simulink model "dynamicInversionControl"  (R2025a)
settings: Solver=FixedStepAuto  StartTime=0.0  StopTime=100  FixedStep=0.01  MaxStep=0.2  RelTol=1e-3
PreLoadFcn:
  | addpath('utils','userDefined');
InitFcn:
  | initialParameters;
values from neighbouring files (symbols this model uses):
  ics = JsonLoad('initialConditions.json')    [initialParameters.m]
  params = JsonLoad('params.json')    [initialParameters.m]
undefined symbols (not defined in the file or in its folder): sim_
libraries: sharedutil x2, aerolibutil x1, dspinverses x1
CloseFcn:
  | rmpath('utils','userDefined');
settings Model: Creator=Cindio  LastModifiedBy=cfeng
settings DebuggingCC: UnconnectedInputMsg=warning  UnconnectedOutputMsg=warning  UnconnectedLineMsg=warning
settings ModelReferenceCC: EnableRefExpFcnMdlSchedulingChecks=on
settings RTWCC: GPUComputeCapability=3.5  DLArmComputeVersion=19.05

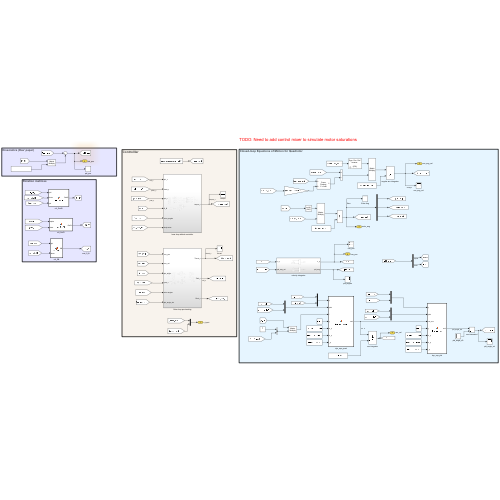
[thumbnail: Simulink's stored preview of the top-level diagram]
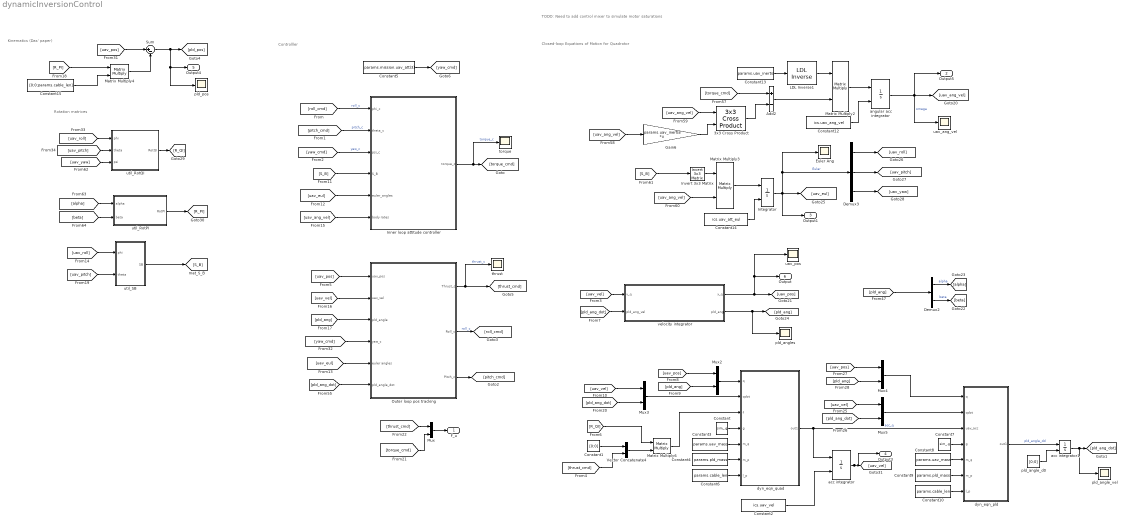
== system dynamicInversionControl ==
  note: TODO: Need to add control mixer to simulate motor saturations
  note: Kinematics (Das' paper)
  note: Controlller
  note: Rotation matrices
  note: Closed-loop Equations of Motion for Quadrotor
  3x3 Cross Product : sharedutil/3x3 Cross Product  aMode=aMode
  Add2 : Sum  Inputs=+-
  Constant : Constant  Value=sim_.g
  Constant1 : Constant  Value=[0;0]  VectorParams1D=off
  Constant10 : Constant  Value=params.cable_len
  Constant12 : Constant  Value=ics.uav_ang_vel  VectorParams1D=off
  Constant13 : Constant  Value=params.uav_inertia
  Constant14 : Constant  Value=ics.uav_att_eul  VectorParams1D=off
  Constant15 : Constant  Value=[0;0;params.cable_len]  VectorParams1D=off
  Constant2 : Constant  Value=ics.uav_vel  VectorParams1D=off
  Constant3 : Constant  Value=params.uav_mass
  Constant4 : Constant  Value=params.pld_mass
  Constant5 : Constant  Value=params.mission.uav_att(3)
  Constant6 : Constant  Value=params.cable_len
  Constant7 : Constant  Value=sim_.g
  Constant8 : Constant  Value=params.uav_mass
  Constant9 : Constant  Value=params.pld_mass
  Demux2 : Demux  Outputs=2
  Demux3 : Demux  Outputs=3
  Euler Ang : Scope
      settings: ActiveDisplayYMinimum=-0.7197540359102037  ActiveDisplayYMaximum=0.7012052127427264  DataLoggingVariableName=ScopeData2
  Gain6 : Gain  Gain=params.uav_inertia  Multiplication=Matrix(K*u)
  Inner loop attitude controller : Subsystem
  Integrator : Integrator  InitialConditionSource=external
  Invert 3x3 Matrix : aerolibutil/Invert  3x3 Matrix
  LDL Inverse1 : dspinverses/LDL Inverse  errmode=Error
  Matrix Multiply{2..4,6} (4 alike) : Product  Multiplication=Matrix(*)
  Mux{,2..5} (5 alike) : Mux  Inputs=2
  Outer loop pos tracking : Subsystem
  Sum : Sum  Inputs=|+-
  Vector Concatenate4 : Concatenate
  acc integrator : Integrator  InitialConditionSource=external
  acc integrator1 : Integrator  InitialConditionSource=external
  angular acc integrator : Integrator  InitialConditionSource=external
  dyn_eqn_pld : MATLAB Function  TreatAsAtomicUnit=on
  dyn_eqn_quad : MATLAB Function  TreatAsAtomicUnit=on
  pld_angle_d0 : Constant  Value=[0;0]  VectorParams1D=off
  pld_angle_vel : Scope
      settings: ActiveDisplayYMinimum=-0.01918  ActiveDisplayYMaximum=0.02061
  pld_angles : Scope
      settings: ActiveDisplayYMinimum=-53.3982088920729  ActiveDisplayYMaximum=39.179802985091776  DataLoggingVariableName=ScopeData3
  pld_pos : Scope
      settings: ActiveDisplayYMinimum=-0.94357  ActiveDisplayYMaximum=8.49211  DataLoggingVariableName=ScopeData3
  thrust : Scope
      settings: ActiveDisplayYMinimum=3.473159317161512  ActiveDisplayYMaximum=9.47908451766764
  torque : Scope
      settings: ActiveDisplayYMinimum=-0.02838  ActiveDisplayYMaximum=0.01772  YLabel=rad
  uav_ang_vel : Scope
      settings: Title=UAV Angular Velocity  ActiveDisplayYMinimum=-0.61468  ActiveDisplayYMaximum=0.88244  YLabel=rad/s
  uav_pos : Scope
      settings: Title=UAV Position  ActiveDisplayYMinimum=-0.93903  ActiveDisplayYMaximum=8.45126  YLabel=position (m)  DataLoggingVariableName=ScopeData4
  util_RotPI : MATLAB Function  TreatAsAtomicUnit=on
  util_RotQI : MATLAB Function  TreatAsAtomicUnit=on
  util_SB : MATLAB Function  TreatAsAtomicUnit=on
  velocity integrator : Subsystem
  F_u : Outport  SignalName=u_input
  Output5 : Outport  Port=2  SignalName=uav_ang_vel
  Output1 : Outport  Port=3  SignalName=euler_ang
  Output3 : Outport  Port=4  SignalName=uav_vel
  Output4 : Outport  Port=5  SignalName=pld_pos
  Output : Outport  Port=6  SignalName=uav_pos
  wires:
  [roll_cmd] -> Inner loop attitude controller/1(phi_c)  "roll_c"
  [pitch_cmd] -> Inner loop attitude controller/2(theta_c)  "pitch_c"
  [yaw_cmd] -> Inner loop attitude controller/3(psi_c)  "yaw_c"
  [S_B] -> Inner loop attitude controller/4(S_B)
  [uav_ang_vel] -> Inner loop attitude controller/6(body rates)
  Inner loop attitude controller/1(torque_c) -> torque/1, [torque_cmd]  "torque_c"
  [uav_pos] -> Outer loop pos tracking/1(uav_pos)
  [uav_vel] -> Outer loop pos tracking/2(uav_vel)
  [pld_ang] -> Outer loop pos tracking/3(pld_angle)
  [R_PI] -> Matrix Multiply4/1
  Outer loop pos tracking/3(Pitch_c) -> [pitch_cmd]
  Outer loop pos tracking/2(Roll_c) -> [roll_cmd]  "roll_c"
  Matrix Multiply4/1 -> Sum/2
  Sum/1 -> pld_pos/1, Output4/1, [pld_pos]
  [uav_pos] -> Sum/1
  [yaw_cmd] -> Outer loop pos tracking/4(yaw_c)
  [uav_eul] -> Outer loop pos tracking/5(euler angles)
  Constant5/1 -> [yaw_cmd]
  [pld_ang] -> Demux2/1
  Demux2/2 -> [beta]  "beta"
  Demux2/1 -> [alpha]  "alpha"
  [pld_ang_dot] -> Outer loop pos tracking/6(pld_angle_dot)
  LDL Inverse1/1 -> Matrix Multiply2/1
  angular acc integrator/1 -> Output5/1, [uav_ang_vel], uav_ang_vel/1  "omega"
  Constant12/1 -> angular acc integrator/2
  Matrix Multiply2/1 -> angular acc integrator/1
  Constant13/1 -> LDL Inverse1/1
  Add2/1 -> Matrix Multiply2/2
  [torque_cmd] -> Add2/1
  [uav_ang_vel] -> Gain6/1
  Gain6/1 -> 3x3 Cross Product/2
  [uav_ang_vel] -> 3x3 Cross Product/1
  3x3 Cross Product/1 -> Add2/2
  [S_B] -> Invert 3x3 Matrix/1
  [uav_ang_vel] -> Matrix Multiply3/2
  Invert 3x3 Matrix/1 -> Matrix Multiply3/1
  Matrix Multiply3/1 -> Integrator/1
  Constant14/1 -> Integrator/2
  Integrator/1 -> Output1/1, Demux3/1, Euler Ang/1, [uav_eul]  "Euler"
  Demux3/1 -> [uav_roll]
  Demux3/3 -> [uav_yaw]
  Demux3/2 -> [uav_pitch]
  [uav_eul] -> Inner loop attitude controller/5(euler_angles)
  Constant15/1 -> Matrix Multiply4/2
  Outer loop pos tracking/1(Thrust_c) -> [thrust_cmd], thrust/1  "thrust_c"
  [uav_roll] -> util_RotQI/1(phi)
  [uav_pitch] -> util_RotQI/2(theta)
  [uav_yaw] -> util_RotQI/3(psi)
  [alpha] -> util_RotPI/1(alpha)
  [beta] -> util_RotPI/2(beta)
  util_RotQI/1(RotQI) -> [R_QI]
  util_RotPI/1(RotPI) -> [R_PI]
  [uav_roll] -> util_SB/1(phi)
  [uav_pitch] -> util_SB/2(theta)
  util_SB/1(SB) -> [S_B]
  Constant2/1 -> acc integrator/2
  dyn_eqn_quad/1(out1) -> dyn_eqn_pld/3(uav_acc), acc integrator/1  "acc_q"
  Constant1/1 -> Vector Concatenate4/1
  [R_QI] -> Matrix Multiply6/1
  Vector Concatenate4/1 -> Matrix Multiply6/2
  [thrust_cmd] -> Vector Concatenate4/2
  Matrix Multiply6/1 -> dyn_eqn_quad/3(f)
  velocity integrator/2(pld_ang) -> pld_angles/1, [pld_ang]
  dyn_eqn_pld/1(out1) -> acc integrator1/1  "pld_angle_dd"
  acc integrator1/1 -> pld_angle_vel/1, [pld_ang_dot]
  [uav_vel] -> velocity integrator/1(v_q)
  [pld_ang_dot] -> velocity integrator/2(pld_ang_vel)
  [uav_pos] -> Mux2/1
  [uav_vel] -> Mux3/1
  [pld_ang] -> Mux2/2
  [pld_ang_dot] -> Mux3/2
  acc integrator/1 -> Output3/1, [uav_vel]
  velocity integrator/1(x_q) -> uav_pos/1, Output/1, [uav_pos]
  Mux3/1 -> dyn_eqn_quad/2(qdot)
  Mux2/1 -> dyn_eqn_quad/1(q)
  [pld_ang_dot] -> Mux5/2
  [uav_pos] -> Mux4/1
  [uav_vel] -> Mux5/1
  Mux5/1 -> dyn_eqn_pld/2(qdot)
  Mux4/1 -> dyn_eqn_pld/1(q)
  [pld_ang] -> Mux4/2
  pld_angle_d0/1 -> acc integrator1/2
  [thrust_cmd] -> Mux/1
  [torque_cmd] -> Mux/2
  Mux/1 -> F_u/1
  Constant/1 -> dyn_eqn_quad/4(g)
  Constant3/1 -> dyn_eqn_quad/5(m_q)
  Constant4/1 -> dyn_eqn_quad/6(m_p)
  Constant6/1 -> dyn_eqn_quad/7(l_p)
  Constant9/1 -> dyn_eqn_pld/6(m_p)
  Constant7/1 -> dyn_eqn_pld/4(g)
  Constant8/1 -> dyn_eqn_pld/5(m_q)
  Constant10/1 -> dyn_eqn_pld/7(l_p)

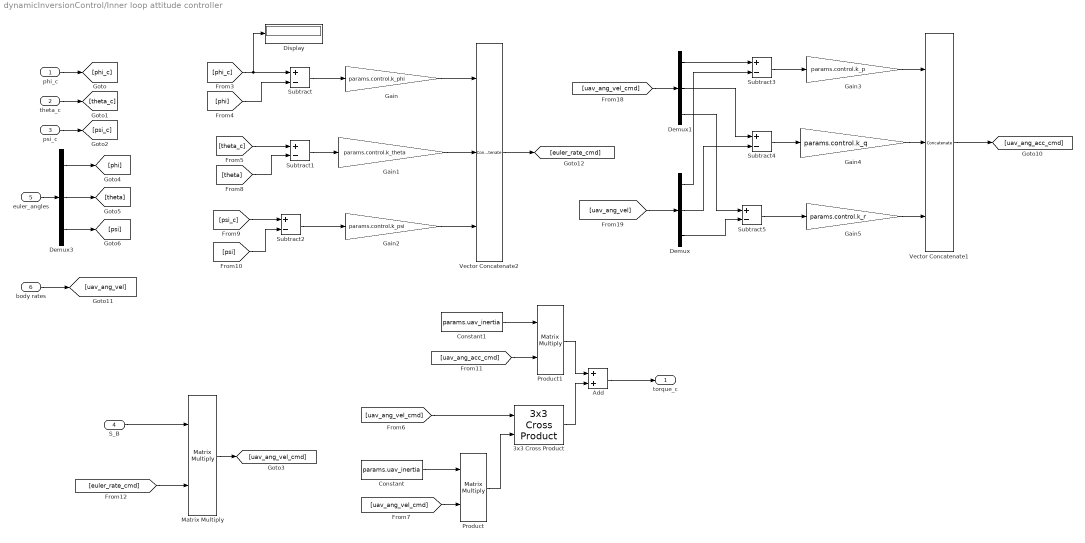
== system dynamicInversionControl/Inner loop attitude controller ==
  phi_c : Inport
  theta_c : Inport  Port=2
  psi_c : Inport  Port=3
  S_B : Inport  Port=4
  euler_angles : Inport  Port=5
  body rates : Inport  Port=6
  3x3 Cross Product : sharedutil/3x3 Cross Product  aMode=aMode
  Add : Sum
  Constant : Constant  Value=params.uav_inertia
  Constant1 : Constant  Value=params.uav_inertia
  Demux : Demux  Outputs=3
  Demux1 : Demux  Outputs=3
  Demux3 : Demux  Outputs=3
  Display : Display
  Gain : Gain  Gain=params.control.k_phi
  Gain1 : Gain  Gain=params.control.k_theta
  Gain2 : Gain  Gain=params.control.k_psi
  Gain3 : Gain  Gain=params.control.k_p
  Gain4 : Gain  Gain=params.control.k_q
  Gain5 : Gain  Gain=params.control.k_r
  Matrix Multiply : Product  Multiplication=Matrix(*)
  Product : Product  Multiplication=Matrix(*)
  Product1 : Product  Multiplication=Matrix(*)
  Subtract{,1..5} (6 alike) : Sum  Inputs=+-
  Vector Concatenate1 : Concatenate  NumInputs=3  Mode=Multidimensional array
  Vector Concatenate2 : Concatenate  NumInputs=3  Mode=Multidimensional array
  torque_c : Outport
  wires:
  phi_c/1 -> [phi_c]
  theta_c/1 -> [theta_c]
  psi_c/1 -> [psi_c]
  S_B/1 -> Matrix Multiply/1
  Constant/1 -> Product/1
  Matrix Multiply/1 -> [uav_ang_vel_cmd]
  Product/1 -> 3x3 Cross Product/2
  [uav_ang_vel_cmd] -> 3x3 Cross Product/1
  [uav_ang_vel_cmd] -> Product/2
  3x3 Cross Product/1 -> Add/2
  Add/1 -> torque_c/1
  euler_angles/1 -> Demux3/1
  Constant1/1 -> Product1/1
  Product1/1 -> Add/1
  [phi] -> Subtract/2
  [phi_c] -> Display/1, Subtract/1
  [theta_c] -> Subtract1/1
  [theta] -> Subtract1/2
  [psi_c] -> Subtract2/1
  [psi] -> Subtract2/2
  Subtract/1 -> Gain/1
  Subtract1/1 -> Gain1/1
  Subtract2/1 -> Gain2/1
  [uav_ang_acc_cmd] -> Product1/2
  Gain/1 -> Vector Concatenate2/1
  Gain1/1 -> Vector Concatenate2/2
  Gain2/1 -> Vector Concatenate2/3
  Subtract3/1 -> Gain3/1
  Gain4/1 -> Vector Concatenate1/2
  Subtract5/1 -> Gain5/1
  Gain5/1 -> Vector Concatenate1/3
  Gain3/1 -> Vector Concatenate1/1
  Subtract4/1 -> Gain4/1
  Vector Concatenate1/1 -> [uav_ang_acc_cmd]
  [uav_ang_vel_cmd] -> Demux1/1
  body rates/1 -> [uav_ang_vel]
  [uav_ang_vel] -> Demux/1
  Demux1/1 -> Subtract3/1
  Demux/1 -> Subtract3/2
  Demux1/2 -> Subtract4/1
  Demux1/3 -> Subtract5/1
  Demux/2 -> Subtract4/2
  Demux/3 -> Subtract5/2
  Vector Concatenate2/1 -> [euler_rate_cmd]
  [euler_rate_cmd] -> Matrix Multiply/2
  Demux3/2 -> [theta]
  Demux3/3 -> [psi]
  Demux3/1 -> [phi]

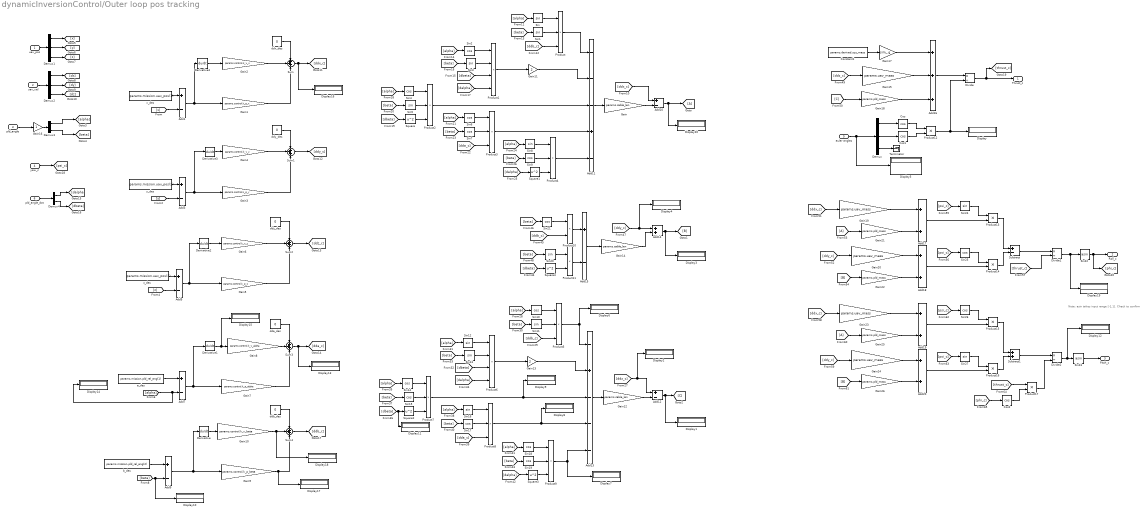
== system dynamicInversionControl/Outer loop pos tracking ==
  note: Note: asin takes input range [-1,1]. Check to confirm
  uav_pos : Inport
  uav_vel : Inport  Port=2
  pld_angle : Inport  Port=3
  yaw_c : Inport  Port=4
  euler angles : Inport  Port=5
  pld_angle_dot : Inport  Port=6
  Add{1,3,5,7,9..10,12,15} (8 alike) : Sum  Inputs=+-
  Add11 : Sum  Inputs=---+-
  Add13 : Sum  Inputs=-+---
  Add{14,17..20} (5 alike) : Sum
  Add16 : Sum  Inputs=+++
  Constant1 : Constant  Value=params.derived.sys_mass
  Cos : Trigonometry  Operator=cos
  Cos1 : Trigonometry  Operator=cos
  Cos2 : Trigonometry  Operator=cos
  Demux : Demux  Outputs=3
  Demux1 : Demux  Outputs=3
  Demux2 : Demux  Outputs=3
  Demux3 : Demux  Outputs=2
  Demux4 : Demux  Outputs=2
  Derivative{,1..4} (5 alike) : Derivative
  Display{,1..20} (21 alike) : Display
  Divide : Product  Inputs=*/
  Divide1 : Product  Inputs=*/
  Divide2 : Product  Inputs=*/
  From53 : From
  From60 : From
  Gain : Gain  Gain=params.cable_len
  Gain1 : Gain  Gain=params.control.k_p_x
  Gain10 : Gain  Gain=params.control.k_v_beta
  Gain11 : Gain  Gain=2
  Gain12 : Gain  Gain=params.cable_len
  Gain13 : Gain  Gain=2
  Gain14 : Gain  Gain=params.cable_len
  Gain{15,19..20,23..24} (5 alike) : Gain  Gain=params.uav_mass
  Gain16 : Gain
  Gain17 : Gain  Gain=sim_.g
  Gain{18,21..22,25..26} (5 alike) : Gain  Gain=params.pld_mass
  Gain2 : Gain  Gain=params.control.k_v_x
  Gain3 : Gain  Gain=params.control.k_p_y
  Gain4 : Gain  Gain=params.control.k_v_y
  Gain5 : Gain  Gain=params.control.k_p_z
  Gain6 : Gain  Gain=params.control.k_v_z
  Gain7 : Gain  Gain=params.control.k_p_alpha
  Gain8 : Gain  Gain=params.control.k_v_alpha
  Gain9 : Gain  Gain=params.control.k_p_beta
  Goto : Goto
  Product{,2..5,7..9} (8 alike) : Product  Inputs=3
  Product1 : Product  Inputs=4
  Product{10..17} (8 alike) : Product
  Product6 : Product  Inputs=4
  Sin{,1,3,5,8,11..13,16,20,24,27} (12 alike) : Trigonometry  OutputSignalType=real
  Sin{2,4,6..7,9..10,14..15,17..19,21,25..26} (14 alike) : Trigonometry  Operator=cos  OutputSignalType=real
  Sin22 : Trigonometry  Operator=asin  OutputSignalType=real
  Sin23 : Trigonometry  Operator=asin  OutputSignalType=real
  Square{,1..4} (5 alike) : Math  Operator=square
  Subtract : Sum  Inputs=+-
  Subtract1 : Sum
  Sum{,1..4} (5 alike) : Sum  Inputs=+++
  Terminator : Terminator
  a_des : Constant  Value=params.mission.pld_rel_ang(1)
  b_des : Constant  Value=params.mission.pld_rel_ang(2)
  dda_des : Constant  Value=0
  ddb_des : Constant  Value=0
  ddx_des : Constant  Value=0
  ddy_des : Constant  Value=0
  ddz_des : Constant  Value=0
  x_des : Constant  Value=params.mission.uav_pos(1)
  y_des : Constant  Value=params.mission.uav_pos(2)
  z_des : Constant  Value=params.mission.uav_pos(3)
  Thrust_c : Outport
  Roll_c : Outport  Port=2
  Pitch_c : Outport  Port=3
  wires:
  uav_pos/1 -> Demux1/1
  uav_vel/1 -> Demux2/1
  pld_angle/1 -> Gain16/1
  Demux3/1 -> [alpha]
  Demux3/2 -> [beta]
  Demux1/1 -> [x]
  Demux1/2 -> [y]
  Demux1/3 -> [z]
  Demux2/2 -> [dy]
  Demux2/3 -> [dz]
  Demux2/1 -> [dx]
  [x] -> Add1/2
  Gain2/1 -> Sum/2
  Add1/1 -> Derivative4/1, Gain1/1
  Gain1/1 -> Sum/3
  x_des/1 -> Add1/1
  ddx_des/1 -> Sum/1
  Sum/1 -> Display16/1, [ddx_c]
  Sum1/1 -> [ddy_c]
  Add3/1 -> Derivative3/1, Gain3/1
  y_des/1 -> Add3/1
  Gain4/1 -> Sum1/2
  ddy_des/1 -> Sum1/1
  [y] -> Add3/2
  Gain3/1 -> Sum1/3
  Sum2/1 -> [ddz_c]
  ddz_des/1 -> Sum2/1
  Gain5/1 -> Sum2/3
  z_des/1 -> Add5/1
  Gain6/1 -> Sum2/2
  [z] -> Add5/2
  Add5/1 -> Derivative2/1, Gain5/1
  Sum3/1 -> Display13/1, [dda_c]
  dda_des/1 -> Sum3/1
  Gain7/1 -> Sum3/3
  a_des/1 -> Add7/1
  Gain8/1 -> Sum3/2
  [alpha] -> Display14/1, Add7/2
  Add7/1 -> Derivative1/1, Gain7/1
  Add9/1 -> Gain9/1, Derivative/1
  [beta] -> Display10/1, Add9/2
  Gain10/1 -> Display18/1, Sum4/2
  ddb_des/1 -> Sum4/1
  Gain9/1 -> Display17/1, Sum4/3
  Sum4/1 -> [ddb_c]
  b_des/1 -> Add9/1
  Add11/1 -> Gain/1
  Gain/1 -> Add10/2
  [ddx_c] -> Add10/1
  Add10/1 -> Display20/1, Goto/1
  [alpha] -> Sin/1
  [beta] -> Sin1/1
  Sin/1 -> Product/1
  Sin1/1 -> Product/2
  [ddb_c] -> Product/3
  Product/1 -> Add11/1
  Sin2/1 -> Product1/1
  [dbeta] -> Product1/3
  [beta] -> Sin3/1
  [alpha] -> Sin2/1
  Sin3/1 -> Product1/2
  Product1/1 -> Gain11/1
  [dalpha] -> Product1/4
  Product2/1 -> Add11/3
  Sin4/1 -> Product2/1
  [dbeta] -> Square/1
  [beta] -> Sin5/1
  [alpha] -> Sin4/1
  Sin5/1 -> Product2/2
  Square/1 -> Product2/3
  Product3/1 -> Add11/4
  Sin6/1 -> Product3/1
  [dda_c] -> Product3/3
  [beta] -> Sin7/1
  [alpha] -> Sin6/1
  Sin7/1 -> Product3/2
  Product4/1 -> Add11/5
  Sin8/1 -> Product4/1
  [dalpha] -> Square1/1
  [beta] -> Sin9/1
  [alpha] -> Sin8/1
  Sin9/1 -> Product4/2
  Square1/1 -> Product4/3
  Gain11/1 -> Add11/2
  Sin17/1 -> Product8/2
  [ddz_c] -> Display2/1, Add12/1
  [dda_c] -> Product8/3
  [beta] -> Sin19/1
  [dbeta] -> Display11/1, Square2/1
  Sin18/1 -> Product9/1
  Square2/1 -> Product7/3
  Product5/1 -> Add13/1, Display6/1
  Product9/1 -> Display7/1, Add13/5
  [beta] -> Sin11/1
  [beta] -> Sin17/1
  [alpha] -> Sin12/1
  Sin16/1 -> Product8/1
  Sin12/1 -> Product6/1
  [beta] -> Sin13/1
  Product8/1 -> Display8/1, Add13/4
  Sin14/1 -> Product7/1
  Sin13/1 -> Product6/2
  Gain13/1 -> Add13/2
  [dbeta] -> Product6/3
  Square3/1 -> Product9/3
  [alpha] -> Sin18/1
  [ddb_c] -> Product5/3
  Product7/1 -> Display9/1, Add13/3
  [dalpha] -> Product6/4
  Sin10/1 -> Product5/1
  [dalpha] -> Square3/1
  Sin15/1 -> Product7/2
  [alpha] -> Sin14/1
  Add13/1 -> Gain12/1
  Product6/1 -> Gain13/1
  Sin11/1 -> Product5/2
  [beta] -> Sin15/1
  Gain12/1 -> Add12/2
  Sin19/1 -> Product9/2
  [alpha] -> Sin16/1
  [alpha] -> Sin10/1
  Add12/1 -> Display1/1, [C]
  Sin21/1 -> Product10/1
  [beta] -> Sin21/1
  [ddb_c] -> Product10/2
  [ddy_c] -> Display4/1, Add14/1
  Gain14/1 -> Add14/2
  Add15/1 -> Gain14/1
  Add14/1 -> Display3/1, [B]
  Product10/1 -> Add15/1
  [beta] -> Sin20/1
  Sin20/1 -> Product11/1
  [dbeta] -> Square4/1
  Square4/1 -> Product11/2
  Product11/1 -> Add15/2
  [ddz_c] -> Gain15/1
  Constant1/1 -> Gain17/1
  [C] -> Gain18/1
  Gain17/1 -> Add16/1
  Gain15/1 -> Add16/2
  Gain18/1 -> Add16/3
  Add16/1 -> Divide/1
  Divide/1 -> [thrust_c], Thrust_c/1
  Cos/1 -> Product12/1
  Cos1/1 -> Product12/2
  Product12/1 -> Divide/2, Display/1
  Demux/2 -> Cos1/1
  euler angles/1 -> Display5/1, Demux/1
  yaw_c/1 -> [psi_c]
  Sin22/1 -> [phi_c], Roll_c/1
  Sin23/1 -> Pitch_c/1
  [ddx_c] -> Gain19/1
  [ddy_c] -> Gain20/1
  From53/1 -> Gain21/1
  [B] -> Gain22/1
  Gain19/1 -> Add17/1
  Gain21/1 -> Add17/2
  Gain20/1 -> Add18/1
  Gain22/1 -> Add18/2
  [psi_c] -> Sin24/1
  Sin24/1 -> Product13/1
  Add17/1 -> Product13/2
  Sin25/1 -> Product14/1
  Add18/1 -> Product14/2
  [psi_c] -> Sin25/1
  Product14/1 -> Subtract/2
  Product13/1 -> Subtract/1
  Subtract/1 -> Divide1/1
  [thrust_c] -> Divide1/2
  Divide1/1 -> Display19/1, Sin22/1
  From60/1 -> Gain25/1
  [ddy_c] -> Gain24/1
  Sin26/1 -> Product15/1
  Gain26/1 -> Add20/2
  Gain25/1 -> Add19/2
  Add19/1 -> Product15/2
  Divide2/1 -> Display12/1, Sin23/1
  Product16/1 -> Subtract1/2
  Gain23/1 -> Add19/1
  Subtract1/1 -> Divide2/1
  [thrust_c] -> Product17/1
  Product15/1 -> Subtract1/1
  Add20/1 -> Product16/2
  [B] -> Gain26/1
  Gain24/1 -> Add20/1
  [psi_c] -> Sin27/1
  Sin27/1 -> Product16/1
  [ddx_c] -> Gain23/1
  [psi_c] -> Sin26/1
  Product17/1 -> Divide2/2
  [phi_c] -> Cos2/1
  Cos2/1 -> Product17/2
  pld_angle_dot/1 -> Demux4/1
  Demux4/1 -> [dalpha]
  Demux4/2 -> [dbeta]
  Demux/1 -> Cos/1
  Demux/3 -> Terminator/1
  Derivative/1 -> Gain10/1
  Derivative1/1 -> Display15/1, Gain8/1
  Derivative4/1 -> Gain2/1
  Derivative3/1 -> Gain4/1
  Derivative2/1 -> Gain6/1
  Gain16/1 -> Demux3/1

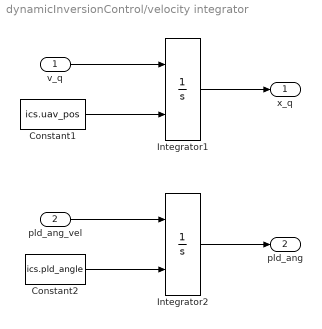
== system dynamicInversionControl/velocity integrator ==
  v_q : Inport
  pld_ang_vel : Inport  Port=2
  Constant1 : Constant  Value=ics.uav_pos
  Constant2 : Constant  Value=ics.pld_angle
  Integrator1 : Integrator  InitialConditionSource=external
  Integrator2 : Integrator  InitialConditionSource=external
  x_q : Outport
  pld_ang : Outport  Port=2
  wires:
  Constant1/1 -> Integrator1/2
  v_q/1 -> Integrator1/1
  Integrator1/1 -> x_q/1
  Constant2/1 -> Integrator2/2
  Integrator2/1 -> pld_ang/1
  pld_ang_vel/1 -> Integrator2/1

== matlab function dynamicInversionControl/util_RotPI ==
  data: alpha input; RotPI output; beta input
function RotPI = util_RotPI(alpha, beta)
% Rotation Matrix:
%   Functionality    : Called to convert translations from  
%                      payload frame to inertial frame
%   Inputs           : Payload angles
%   Outputs          : Rotation matrix

RotPI = [cos(alpha)  sin(alpha)*sin(beta) sin(alpha)*cos(beta);
                  0             cos(beta)           -sin(beta);
         -sin(alpha) cos(alpha)*sin(beta) cos(alpha)*cos(beta)];

== matlab function dynamicInversionControl/util_RotQI ==
  data: phi input; RotQI output; theta input; psi input
function RotQI = util_RotQI(phi,theta,psi)
% Rotation Matrix:
%   Functionality    : Called to convert translations from  
%                      body frame to inertial frame
%   Inputs           : Euler angles
%   Outputs          : Rotation matrix
RotQI = [cos(theta)*cos(psi) sin(phi)*sin(theta)*cos(psi)-cos(phi)*sin(psi) cos(phi)*sin(theta)*cos(psi)+sin(phi)*sin(psi);
         cos(theta)*sin(psi) sin(phi)*sin(theta)*sin(psi)+cos(phi)*cos(psi) cos(phi)*sin(theta)*sin(psi)-sin(phi)*cos(psi);
         -sin(theta) sin(phi)*cos(theta) cos(phi)*cos(theta)];

== matlab function dynamicInversionControl/util_SB ==
  data: phi input; SB output; theta input
function SB = util_RotPI(phi,theta)
% Rotation Matrix:
%   Functionality    : Transforms Euler rates to body rates 
%   Inputs           : Euler angles
%   Outputs          : Matrix to get angular velocities

SB = [1            0             -sin(theta);
      0      cos(phi)    cos(theta)*sin(phi);
      0     -sin(phi)    cos(phi)*cos(theta)];

== matlab function dynamicInversionControl/dyn_eqn_quad ==
  data: q input; out1 output; qdot input; f input; g input; m_q input; m_p input; l_p input
function out1 = dyn_eqn_quad(q,qdot,f,g,m_q,m_p,l_p)
%DYN_EQN_QUAD
%    OUT1 = DYN_EQN_QUAD(X_S1,X_S2,X_S3,X_S4,X_S5,V_S1,V_S2,V_S3,V_S4,V_S5,F_L1,F_L2,F_L3,G,L_P,M_P,M_Q)

%    This function was generated by the Symbolic Math Toolbox version 8.7.
%    03-Sep-2022 18:10:28

x_s1 = q(1);
x_s2 = q(2);
x_s3 = q(3);
x_s4 = q(4);
x_s5 = q(5);
v_s1 = qdot(1);
v_s2 = qdot(2);
v_s3 = qdot(3);
v_s4 = qdot(4);
v_s5 = qdot(5);
F_l1 = f(1);
F_l2 = f(2);
F_l3 = f(3);

t2 = cos(x_s4);
t3 = cos(x_s5);
t4 = sin(x_s4);
t5 = sin(x_s5);
t6 = m_p+m_q;
t7 = v_s4.^2;
t8 = v_s5.^2;
t9 = 1.0./t6;
out1 = [-t9.*(-F_l1+l_p.*m_p.*t3.*t4.*t7+l_p.*m_p.*t3.*t4.*t8+l_p.*m_p.*t2.*t5.*v_s4.*v_s5.*2.0);t9.*(F_l2+l_p.*m_p.*t5.*t8);-t9.*(-F_l3+g.*m_p+g.*m_q+l_p.*m_p.*t2.*t3.*t7+l_p.*m_p.*t2.*t3.*t8-l_p.*m_p.*t4.*t5.*v_s4.*v_s5.*2.0)];

== matlab function dynamicInversionControl/dyn_eqn_pld ==
  data: q input; out1 output; qdot input; uav_acc input; g input; m_q input; m_p input; l_p input
function out1 = dyn_eqn_pld(q, qdot, uav_acc,g,m_q,m_p,l_p)
%DYN_EQN_PLD
%    OUT1 = DYN_EQN_PLD(X_S1,X_S2,X_S3,X_S4,X_S5,V_S1,V_S2,V_S3,V_S4,V_S5,A_Q1,A_Q2,A_Q3,G,L_P,M_P,M_Q)

%    This function was generated by the Symbolic Math Toolbox version 8.7.
%    03-Sep-2022 18:10:28

x_s1 = q(1);
x_s2 = q(2);
x_s3 = q(3);
x_s4 = q(4);
x_s5 = q(5);
v_s1 = qdot(1);
v_s2 = qdot(2);
v_s3 = qdot(3);
v_s4 = qdot(4);
v_s5 = qdot(5);
a_q1 = uav_acc(1);
a_q2 = uav_acc(2);
a_q3 = uav_acc(3);

t2 = cos(x_s4);
t3 = cos(x_s5);
t4 = sin(x_s4);
t5 = sin(x_s5);
t6 = 1.0./l_p;
out1 = [(t3.*t6.*(a_q1.*t2-a_q3.*t4-g.*t4+l_p.*t5.*v_s4.*v_s5.*2.0))./(t3.^2+1.0);t6.*(a_q2.*t3+a_q1.*t4.*t5+a_q3.*t2.*t5+g.*t2.*t5+l_p.*t3.*t5.*v_s4.^2).*(-1.0./2.0)];
